simulink model "MIL_ASW"  (R2019b)
settings: Solver=FixedStepDiscrete  StartTime=0.0  StopTime=2  FixedStep=0.001  RelTol=1e-3  EnableMultiTasking=on
model workspace (MAT data in the model file):
  AccPedlCanVal : Simulink.Signal (value not decoded)
  AccPedlVal : Simulink.Signal (value not decoded)
  BrkPedlCanVal : Simulink.Signal (value not decoded)
  BrkPedlVal : Simulink.Signal (value not decoded)
  Cal1 : Simulink.Parameter (value not decoded)
  Cal10 : Simulink.Parameter (value not decoded)
  Cal11 : Simulink.Parameter (value not decoded)
  Cal12 : Simulink.Parameter (value not decoded)
  Cal2 : Simulink.Parameter (value not decoded)
  Cal3 : Simulink.Parameter (value not decoded)
  Cal4 : Simulink.Parameter (value not decoded)
  Cal5 : Simulink.Parameter (value not decoded)
  Cal6 : Simulink.Parameter (value not decoded)
  Cal7 : Simulink.Parameter (value not decoded)
  Cal8 : Simulink.Parameter (value not decoded)
  Cal9 : Simulink.Parameter (value not decoded)
  Clu1Act : Simulink.Signal (value not decoded)
  Clu1PTar : Simulink.Signal (value not decoded)
  Clu1Req : Simulink.Signal (value not decoded)
  Clu1TqTar : Simulink.Signal (value not decoded)
  Clu2Act : Simulink.Signal (value not decoded)
  Clu2PTar : Simulink.Signal (value not decoded)
  Clu2Req : Simulink.Signal (value not decoded)
  Clu2TqTar : Simulink.Signal (value not decoded)
  CluKissPtPLnch : Simulink.Parameter (value not decoded)
  CluOilTRawVal : Simulink.Signal (value not decoded)
  CluOilTVal : Simulink.Signal (value not decoded)
  CluOpenTqRatMax : Simulink.Parameter (value not decoded)
  CluPMap : Simulink.Parameter (value not decoded)
  CluPMax : Simulink.Parameter (value not decoded)
  CluPMaxGear1 : Simulink.Parameter (value not decoded)
  CluPMaxGear2 : Simulink.Parameter (value not decoded)
  CluPMaxGear3 : Simulink.Parameter (value not decoded)
  CluPMaxGear4 : Simulink.Parameter (value not decoded)
  CluPMaxGear5 : Simulink.Parameter (value not decoded)
  CluPMaxGear6 : Simulink.Parameter (value not decoded)
  CluPMaxGearR : Simulink.Parameter (value not decoded)
  CluPMin : Simulink.Parameter (value not decoded)
  CluPosnMax : Simulink.Parameter (value not decoded)
  CluSoln1IRawVal : Simulink.Signal (value not decoded)
  CluSoln1IReq : Simulink.Signal (value not decoded)
  CluSoln1IReqFlg : Simulink.Signal (value not decoded)
  CluSoln1IVal : Simulink.Signal (value not decoded)
  CluSoln1LineI : Simulink.Parameter (value not decoded)
  CluSoln1LineP : Simulink.Parameter (value not decoded)
  CluSoln1Pwm : Simulink.Signal (value not decoded)
  CluSoln2IRawVal : Simulink.Signal (value not decoded)
  CluSoln2IReq : Simulink.Signal (value not decoded)
  CluSoln2IReqFlg : Simulink.Signal (value not decoded)
  CluSoln2IVal : Simulink.Signal (value not decoded)
  CluSoln2LineI : Simulink.Parameter (value not decoded)
  CluSoln2LineP : Simulink.Parameter (value not decoded)
  CluSoln2Pwm : Simulink.Signal (value not decoded)
  CluTqMap : Simulink.Parameter (value not decoded)
  CrnkSpdRawVal : Simulink.Signal (value not decoded)
  CrnkSpdVal : Simulink.Signal (value not decoded)
  Drive_Intensity_Fuzzy : object (value not decoded)
  DrvIntenFzzy : Simulink.LookupTable (value not decoded)
  EngNIdle : Simulink.Parameter (value not decoded)
  EngNIdleMin : Simulink.Parameter (value not decoded)
  EngSpdCanVal : Simulink.Signal (value not decoded)
  EngThrCanVal : Simulink.Signal (value not decoded)
  EngTqAdd : Simulink.Parameter (value not decoded)
  EngTqCanVal : Simulink.Signal (value not decoded)
  EngTqIntvFlg : Simulink.Signal (value not decoded)
  EngTqIntvRat : Simulink.Signal (value not decoded)
  EngTqMapExtChartc : Simulink.Parameter (value not decoded)
  EngTqMapSpdIndx : Simulink.Parameter (value not decoded)
  EngTqMapThrtIndx : Simulink.Parameter (value not decoded)
  EngTqMapTqMax : Simulink.Parameter (value not decoded)
  EngTqMaxNorm : Simulink.Parameter (value not decoded)
  EngTqRef : Simulink.Parameter (value not decoded)
  EvenCluPRawVal : Simulink.Signal (value not decoded)
  EvenCluPVal : Simulink.Signal (value not decoded)
  EvenInpSpdRawVal : Simulink.Signal (value not decoded)
  EvenInpSpdVal : Simulink.Signal (value not decoded)
  FcnCallTime : Simulink.Parameter (value not decoded)
  FinalRat : Simulink.Parameter (value not decoded)
  Fork1A : Simulink.Parameter (value not decoded)
  Fork1Act : Simulink.Signal (value not decoded)
  Fork1B : Simulink.Parameter (value not decoded)
  Fork1DeltaSpdTar : Simulink.Parameter (value not decoded)
  Fork1MaxSpd1A : Simulink.Parameter (value not decoded)
  Fork1MaxSpd1B : Simulink.Parameter (value not decoded)
  Fork1MaxSpd2A : Simulink.Parameter (value not decoded)
  Fork1MaxSpd2B : Simulink.Parameter (value not decoded)
  Fork1PosnA : Simulink.Parameter (value not decoded)
  Fork1PosnB : Simulink.Parameter (value not decoded)
  Fork1PosnMaxSpd1A : Simulink.Parameter (value not decoded)
  Fork1PosnMaxSpd1B : Simulink.Parameter (value not decoded)
  Fork1PosnMaxSpd2A : Simulink.Parameter (value not decoded)
  Fork1PosnMaxSpd2B : Simulink.Parameter (value not decoded)
  Fork1PosnNeut : Simulink.Parameter (value not decoded)
  Fork1PosnNeutA : Simulink.Parameter (value not decoded)
  Fork1PosnNeutB : Simulink.Parameter (value not decoded)
  Fork1PosnRawVal : Simulink.Signal (value not decoded)
  Fork1PosnSyncA : Simulink.Parameter (value not decoded)
  Fork1PosnSyncB : Simulink.Parameter (value not decoded)
  Fork1PosnVal : Simulink.Signal (value not decoded)
  Fork1SyncTar : Simulink.Parameter (value not decoded)
  Fork2A : Simulink.Parameter (value not decoded)
  Fork2Act : Simulink.Signal (value not decoded)
  Fork2B : Simulink.Parameter (value not decoded)
  Fork2DeltaSpdTar : Simulink.Parameter (value not decoded)
  Fork2MaxSpd1A : Simulink.Parameter (value not decoded)
  Fork2MaxSpd1B : Simulink.Parameter (value not decoded)
  Fork2MaxSpd2A : Simulink.Parameter (value not decoded)
  Fork2MaxSpd2B : Simulink.Parameter (value not decoded)
  Fork2PosnA : Simulink.Parameter (value not decoded)
  Fork2PosnB : Simulink.Parameter (value not decoded)
  Fork2PosnMaxSpd1A : Simulink.Parameter (value not decoded)
  Fork2PosnMaxSpd1B : Simulink.Parameter (value not decoded)
  Fork2PosnMaxSpd2A : Simulink.Parameter (value not decoded)
  Fork2PosnMaxSpd2B : Simulink.Parameter (value not decoded)
  Fork2PosnNeut : Simulink.Parameter (value not decoded)
  Fork2PosnNeutA : Simulink.Parameter (value not decoded)
  Fork2PosnNeutB : Simulink.Parameter (value not decoded)
  Fork2PosnRawVal : Simulink.Signal (value not decoded)
  Fork2PosnSyncA : Simulink.Parameter (value not decoded)
  Fork2PosnSyncB : Simulink.Parameter (value not decoded)
  Fork2PosnVal : Simulink.Signal (value not decoded)
  Fork2SyncTar : Simulink.Parameter (value not decoded)
  Fork3A : Simulink.Parameter (value not decoded)
  Fork3Act : Simulink.Signal (value not decoded)
  Fork3B : Simulink.Parameter (value not decoded)
  Fork3DeltaSpdTar : Simulink.Parameter (value not decoded)
  Fork3MaxSpd1A : Simulink.Parameter (value not decoded)
  Fork3MaxSpd1B : Simulink.Parameter (value not decoded)
  Fork3MaxSpd2A : Simulink.Parameter (value not decoded)
  Fork3MaxSpd2B : Simulink.Parameter (value not decoded)
  Fork3PosnA : Simulink.Parameter (value not decoded)
  Fork3PosnB : Simulink.Parameter (value not decoded)
  Fork3PosnMaxSpd1A : Simulink.Parameter (value not decoded)
  Fork3PosnMaxSpd1B : Simulink.Parameter (value not decoded)
  Fork3PosnMaxSpd2A : Simulink.Parameter (value not decoded)
  Fork3PosnMaxSpd2B : Simulink.Parameter (value not decoded)
  Fork3PosnNeut : Simulink.Parameter (value not decoded)
  Fork3PosnNeutA : Simulink.Parameter (value not decoded)
  Fork3PosnNeutB : Simulink.Parameter (value not decoded)
  Fork3PosnRawVal : Simulink.Signal (value not decoded)
  Fork3PosnSyncA : Simulink.Parameter (value not decoded)
  Fork3PosnSyncB : Simulink.Parameter (value not decoded)
  Fork3PosnVal : Simulink.Signal (value not decoded)
  Fork3SyncTar : Simulink.Parameter (value not decoded)
  Fork4A : Simulink.Parameter (value not decoded)
  Fork4Act : Simulink.Signal (value not decoded)
  Fork4B : Simulink.Parameter (value not decoded)
  Fork4DeltaSpdTar : Simulink.Parameter (value not decoded)
  Fork4MaxSpd1A : Simulink.Parameter (value not decoded)
  Fork4MaxSpd1B : Simulink.Parameter (value not decoded)
  Fork4MaxSpd2A : Simulink.Parameter (value not decoded)
  Fork4MaxSpd2B : Simulink.Parameter (value not decoded)
  Fork4PosnA : Simulink.Parameter (value not decoded)
  Fork4PosnB : Simulink.Parameter (value not decoded)
  Fork4PosnMaxSpd1A : Simulink.Parameter (value not decoded)
  Fork4PosnMaxSpd1B : Simulink.Parameter (value not decoded)
  Fork4PosnMaxSpd2A : Simulink.Parameter (value not decoded)
  Fork4PosnMaxSpd2B : Simulink.Parameter (value not decoded)
  Fork4PosnNeut : Simulink.Parameter (value not decoded)
  Fork4PosnNeutA : Simulink.Parameter (value not decoded)
  Fork4PosnNeutB : Simulink.Parameter (value not decoded)
  Fork4PosnRawVal : Simulink.Signal (value not decoded)
  Fork4PosnSyncA : Simulink.Parameter (value not decoded)
  Fork4PosnSyncB : Simulink.Parameter (value not decoded)
  Fork4PosnVal : Simulink.Signal (value not decoded)
  Fork4SyncTar : Simulink.Parameter (value not decoded)
  FrntWhlRd : Simulink.Parameter (value not decoded)
  GearIdx : Simulink.Parameter (value not decoded)
  GearMax : Simulink.Parameter (value not decoded)
  GearRat : Simulink.Parameter (value not decoded)
  Launch_Engage_Fuzzy : object (value not decoded)
  LnchEngmtFzzy : Simulink.LookupTable (value not decoded)
  LubeSolnIRawVal : Simulink.Signal (value not decoded)
  LubeSolnIReq : Simulink.Signal (value not decoded)
  LubeSolnIVal : Simulink.Signal (value not decoded)
  LubeSolnLineI : Simulink.Parameter (value not decoded)
  LubeSolnLineP : Simulink.Parameter (value not decoded)
  LubeSolnPwm : Simulink.Signal (value not decoded)
  MaiLineSolnIRawVal : Simulink.Signal (value not decoded)
  MaiLineSolnIReq : Simulink.Signal (value not decoded)
  MaiLineSolnIVal : Simulink.Signal (value not decoded)
  MaiLineSolnLineI : Simulink.Parameter (value not decoded)
  MaiLineSolnLineP : Simulink.Parameter (value not decoded)
  MaiLineSolnPwm : Simulink.Signal (value not decoded)
  OddCluPRawVal : Simulink.Signal (value not decoded)
  OddCluPVal : Simulink.Signal (value not decoded)
  OddInpSpdRawVal : Simulink.Signal (value not decoded)
  OddInpSpdVal : Simulink.Signal (value not decoded)
  OutpSpdRawVal : Simulink.Signal (value not decoded)
  OutpSpdVal : Simulink.Signal (value not decoded)
  PsnsrLineP : Simulink.Parameter (value not decoded)
  PsnsrLineV : Simulink.Parameter (value not decoded)
  SftLvrCanVal : Simulink.Signal (value not decoded)
  SftLvrCfm : Simulink.Signal (value not decoded)
  SftLvrVal : Simulink.Signal (value not decoded)
  Shaft1GearAct : Simulink.Signal (value not decoded)
  Shaft1GearReq : Simulink.Signal (value not decoded)
  Shaft2GearAct : Simulink.Signal (value not decoded)
  Shaft2GearReq : Simulink.Signal (value not decoded)
  ShiftMux1SwtReq : Simulink.Signal (value not decoded)
  ShiftMux2SwtReq : Simulink.Signal (value not decoded)
  ShiftSdlEcoDwnSeln : Simulink.Parameter (value not decoded)
  ShiftSdlEcoDwnShift : Simulink.Parameter (value not decoded)
  ShiftSdlEcoUpSeln : Simulink.Parameter (value not decoded)
  ShiftSdlEcoUpShift : Simulink.Parameter (value not decoded)
  ShiftSdlPwrDwnSeln : Simulink.Parameter (value not decoded)
  ShiftSdlPwrDwnShift : Simulink.Parameter (value not decoded)
  ShiftSdlPwrUpSeln : Simulink.Parameter (value not decoded)
  ShiftSdlPwrUpShift : Simulink.Parameter (value not decoded)
  ShiftSdlSACDwnSeln : Simulink.Parameter (value not decoded)
  ShiftSdlSACDwnShift : Simulink.Parameter (value not decoded)
  ShiftSdlSACUpSeln : Simulink.Parameter (value not decoded)
  ShiftSdlSACUpShift : Simulink.Parameter (value not decoded)
  ShiftSdlThrPedlIdx : Simulink.Parameter (value not decoded)
  ShiftSoln1IRawVal : Simulink.Signal (value not decoded)
  ShiftSoln1IReq : Simulink.Signal (value not decoded)
  ShiftSoln1IVal : Simulink.Signal (value not decoded)
  ShiftSoln1LineI : Simulink.Parameter (value not decoded)
  ShiftSoln1LineP : Simulink.Parameter (value not decoded)
  ShiftSoln1Pwm : Simulink.Signal (value not decoded)
  ShiftSoln2IRawVal : Simulink.Signal (value not decoded)
  ShiftSoln2IReq : Simulink.Signal (value not decoded)
  ShiftSoln2IVal : Simulink.Signal (value not decoded)
  ShiftSoln2LineI : Simulink.Parameter (value not decoded)
  ShiftSoln2LineP : Simulink.Parameter (value not decoded)
  ShiftSoln2Pwm : Simulink.Signal (value not decoded)
  SolnOutpTRawVal : Simulink.Signal (value not decoded)
  SolnOutpTVal : Simulink.Signal (value not decoded)
  TSnsr1LineR : Simulink.Parameter (value not decoded)
  TSnsr2LineR : Simulink.Parameter (value not decoded)
  TrsmNrGearAct : Simulink.Signal (value not decoded)
  TrsmNrGearReq : Simulink.Signal (value not decoded)
  TrsmNrPreGearAct : Simulink.Signal (value not decoded)
  TrsmNrPreGearReq : Simulink.Signal (value not decoded)
  Tsnsr1LineT : Simulink.Parameter (value not decoded)
  Tsnsr2LineT : Simulink.Parameter (value not decoded)
  VehSpdCanVal : Simulink.Signal (value not decoded)
  VehSpdTrsmEstimd : Simulink.Signal (value not decoded)
  VehSpdVal : Simulink.Signal (value not decoded)
  VlvBodyTRawVal : Simulink.Signal (value not decoded)
  VlvBodyTVal : Simulink.Signal (value not decoded)
symbols that are objects in the model workspace (value not decoded): CluPMap, CluSoln1LineI, CluSoln1LineP, CluSoln2LineI, CluSoln2LineP, CluTqMap, EngNIdle, EngNIdleMin, EngTqMapThrtIndx, EngTqMapTqMax, EngTqMaxNorm, FcnCallTime, FinalRat, Fork1A, Fork1B, Fork1DeltaSpdTar, Fork1PosnA, Fork1PosnB, Fork1PosnMaxSpd1A, Fork1PosnMaxSpd1B, Fork1PosnMaxSpd2A, Fork1PosnMaxSpd2B, Fork1PosnNeut, Fork1PosnNeutA, Fork1PosnNeutB, Fork1PosnSyncA, Fork1PosnSyncB, Fork1SyncTar, Fork2A, Fork2B, Fork2DeltaSpdTar, Fork2PosnA, Fork2PosnB, Fork2PosnMaxSpd1A, Fork2PosnMaxSpd1B, Fork2PosnMaxSpd2A, Fork2PosnMaxSpd2B, Fork2PosnNeut, Fork2PosnNeutA, Fork2PosnNeutB, Fork2PosnSyncA, Fork2PosnSyncB, Fork2SyncTar, Fork3A, Fork3B, Fork3DeltaSpdTar, Fork3PosnA, Fork3PosnB, Fork3PosnMaxSpd1A, Fork3PosnMaxSpd1B, Fork3PosnMaxSpd2A, Fork3PosnMaxSpd2B, Fork3PosnNeut, Fork3PosnNeutA, Fork3PosnNeutB, Fork3PosnSyncA, Fork3PosnSyncB, Fork3SyncTar, Fork4A, Fork4B
undefined symbols (not defined in the file or in its folder): in1, out1
libraries: simulink x44, fuzblock x3
(part 3 of 10)

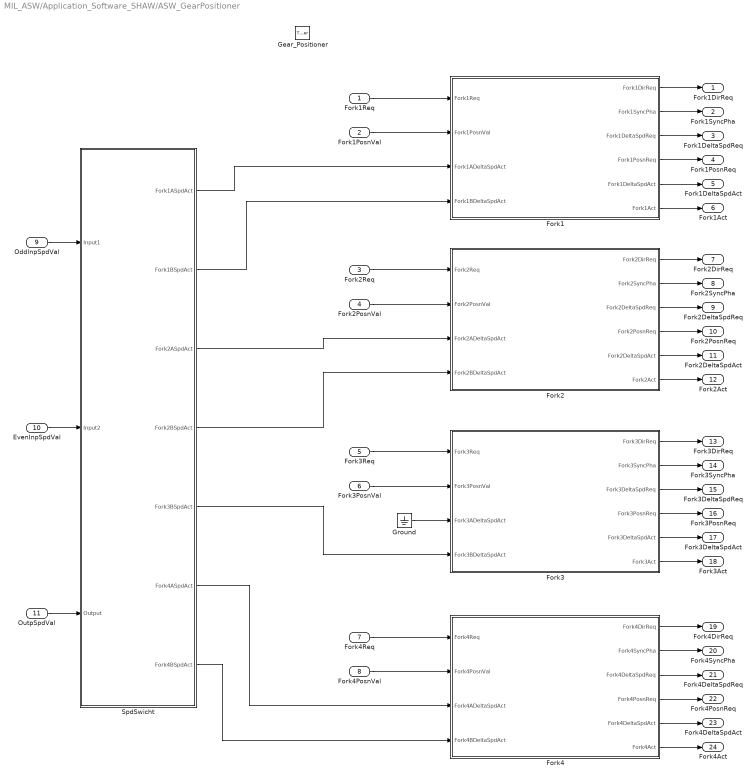
== system MIL_ASW/Application_Software_SHAW/ASW_GearPositioner ==
  Fork1Req : Inport
  Fork1PosnVal : Inport  Port=2
  Fork2Req : Inport  Port=3
  Fork2PosnVal : Inport  Port=4
  Fork3Req : Inport  Port=5
  Fork3PosnVal : Inport  Port=6
  Fork4Req : Inport  Port=7
  Fork4PosnVal : Inport  Port=8
  OddInpSpdVal : Inport  Port=9
  EvenInpSpdVal : Inport  Port=10
  OutpSpdVal : Inport  Port=11
  Gear_Positioner : TriggerPort  TriggerType=function-call  VariantControl=(inherit)  PortDimensions=1
  Fork1 : Stateflow chart  TreatAsAtomicUnit=on
  Fork2 : Stateflow chart  TreatAsAtomicUnit=on
  Fork3 : Stateflow chart  TreatAsAtomicUnit=on
  Fork4 : Stateflow chart  TreatAsAtomicUnit=on
  Ground : Ground
  SpdSwicht : Subsystem
  Fork1DirReq : Outport  VectorParamsAs1DForOutWhenUnconnected=off
  Fork1SyncPha : Outport  Port=2  VectorParamsAs1DForOutWhenUnconnected=off
  Fork1DeltaSpdReq : Outport  Port=3  VectorParamsAs1DForOutWhenUnconnected=off
  Fork1PosnReq : Outport  Port=4  VectorParamsAs1DForOutWhenUnconnected=off
  Fork1DeltaSpdAct : Outport  Port=5  VectorParamsAs1DForOutWhenUnconnected=off
  Fork1Act : Outport  Port=6  VectorParamsAs1DForOutWhenUnconnected=off
  Fork2DirReq : Outport  Port=7  VectorParamsAs1DForOutWhenUnconnected=off
  Fork2SyncPha : Outport  Port=8  VectorParamsAs1DForOutWhenUnconnected=off
  Fork2DeltaSpdReq : Outport  Port=9  VectorParamsAs1DForOutWhenUnconnected=off
  Fork2PosnReq : Outport  Port=10  VectorParamsAs1DForOutWhenUnconnected=off
  Fork2DeltaSpdAct : Outport  Port=11  VectorParamsAs1DForOutWhenUnconnected=off
  Fork2Act : Outport  Port=12  VectorParamsAs1DForOutWhenUnconnected=off
  Fork3DirReq : Outport  Port=13  VectorParamsAs1DForOutWhenUnconnected=off
  Fork3SyncPha : Outport  Port=14  VectorParamsAs1DForOutWhenUnconnected=off
  Fork3DeltaSpdReq : Outport  Port=15  VectorParamsAs1DForOutWhenUnconnected=off
  Fork3PosnReq : Outport  Port=16  VectorParamsAs1DForOutWhenUnconnected=off
  Fork3DeltaSpdAct : Outport  Port=17  VectorParamsAs1DForOutWhenUnconnected=off
  Fork3Act : Outport  Port=18  VectorParamsAs1DForOutWhenUnconnected=off
  Fork4DirReq : Outport  Port=19  VectorParamsAs1DForOutWhenUnconnected=off
  Fork4SyncPha : Outport  Port=20  VectorParamsAs1DForOutWhenUnconnected=off
  Fork4DeltaSpdReq : Outport  Port=21  VectorParamsAs1DForOutWhenUnconnected=off
  Fork4PosnReq : Outport  Port=22  VectorParamsAs1DForOutWhenUnconnected=off
  Fork4DeltaSpdAct : Outport  Port=23  VectorParamsAs1DForOutWhenUnconnected=off
  Fork4Act : Outport  Port=24  VectorParamsAs1DForOutWhenUnconnected=off
  wires:
  SpdSwicht/2(Fork1BSpdAct) -> Fork1/4(Fork1BDeltaSpdAct)
  SpdSwicht/1(Fork1ASpdAct) -> Fork1/3(Fork1ADeltaSpdAct)
  OutpSpdVal/1 -> SpdSwicht/3(Output)
  EvenInpSpdVal/1 -> SpdSwicht/2(Input2)
  OddInpSpdVal/1 -> SpdSwicht/1(Input1)
  Fork4/1(Fork4DirReq) -> Fork4DirReq/1
  Fork4PosnVal/1 -> Fork4/2(Fork4PosnVal)
  Fork4Req/1 -> Fork4/1(Fork4Req)
  Fork4/2(Fork4SyncPha) -> Fork4SyncPha/1
  Fork4/6(Fork4Act) -> Fork4Act/1
  Fork4/3(Fork4DeltaSpdReq) -> Fork4DeltaSpdReq/1
  Fork4/4(Fork4PosnReq) -> Fork4PosnReq/1
  Fork3/1(Fork3DirReq) -> Fork3DirReq/1
  Fork3PosnVal/1 -> Fork3/2(Fork3PosnVal)
  Fork3Req/1 -> Fork3/1(Fork3Req)
  Fork3/2(Fork3SyncPha) -> Fork3SyncPha/1
  Fork3/6(Fork3Act) -> Fork3Act/1
  Fork3/3(Fork3DeltaSpdReq) -> Fork3DeltaSpdReq/1
  Fork3/4(Fork3PosnReq) -> Fork3PosnReq/1
  Fork2/1(Fork2DirReq) -> Fork2DirReq/1
  Fork2PosnVal/1 -> Fork2/2(Fork2PosnVal)
  Fork2Req/1 -> Fork2/1(Fork2Req)
  Fork2/2(Fork2SyncPha) -> Fork2SyncPha/1
  Fork2/6(Fork2Act) -> Fork2Act/1
  Fork2/3(Fork2DeltaSpdReq) -> Fork2DeltaSpdReq/1
  Fork2/4(Fork2PosnReq) -> Fork2PosnReq/1
  Fork1/1(Fork1DirReq) -> Fork1DirReq/1
  Fork1PosnVal/1 -> Fork1/2(Fork1PosnVal)
  Fork1Req/1 -> Fork1/1(Fork1Req)
  Fork1/2(Fork1SyncPha) -> Fork1SyncPha/1
  Fork1/6(Fork1Act) -> Fork1Act/1
  Fork1/3(Fork1DeltaSpdReq) -> Fork1DeltaSpdReq/1
  Fork1/4(Fork1PosnReq) -> Fork1PosnReq/1
  Fork1/5(Fork1DeltaSpdAct) -> Fork1DeltaSpdAct/1
  SpdSwicht/3(Fork2ASpdAct) -> Fork2/3(Fork2ADeltaSpdAct)
  SpdSwicht/4(Fork2BSpdAct) -> Fork2/4(Fork2BDeltaSpdAct)
  Fork2/5(Fork2DeltaSpdAct) -> Fork2DeltaSpdAct/1
  SpdSwicht/5(Fork3BSpdAct) -> Fork3/4(Fork3BDeltaSpdAct)
  Fork3/5(Fork3DeltaSpdAct) -> Fork3DeltaSpdAct/1
  SpdSwicht/6(Fork4ASpdAct) -> Fork4/3(Fork4ADeltaSpdAct)
  SpdSwicht/7(Fork4BSpdAct) -> Fork4/4(Fork4BDeltaSpdAct)
  Fork4/5(Fork4DeltaSpdAct) -> Fork4DeltaSpdAct/1
  Ground/1 -> Fork3/3(Fork3ADeltaSpdAct)

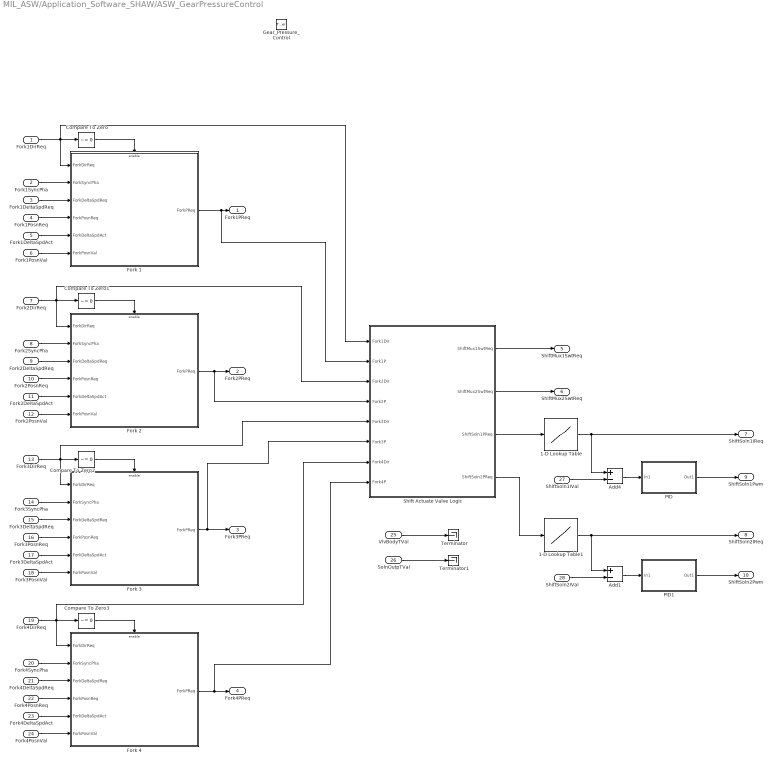
== system MIL_ASW/Application_Software_SHAW/ASW_GearPressureControl ==
  Fork1DirReq : Inport
  Fork1SyncPha : Inport  Port=2
  Fork1DeltaSpdReq : Inport  Port=3
  Fork1PosnReq : Inport  Port=4
  Fork1DeltaSpdAct : Inport  Port=5
  Fork1PosnVal : Inport  Port=6
  Fork2DirReq : Inport  Port=7
  Fork2SyncPha : Inport  Port=8
  Fork2DeltaSpdReq : Inport  Port=9
  Fork2PosnReq : Inport  Port=10
  Fork2DeltaSpdAct : Inport  Port=11
  Fork2PosnVal : Inport  Port=12
  Fork3DirReq : Inport  Port=13
  Fork3SyncPha : Inport  Port=14
  Fork3DeltaSpdReq : Inport  Port=15
  Fork3PosnReq : Inport  Port=16
  Fork3DeltaSpdAct : Inport  Port=17
  Fork3PosnVal : Inport  Port=18
  Fork4DirReq : Inport  Port=19
  Fork4SyncPha : Inport  Port=20
  Fork4DeltaSpdReq : Inport  Port=21
  Fork4PosnReq : Inport  Port=22
  Fork4DeltaSpdAct : Inport  Port=23
  Fork4PosnVal : Inport  Port=24
  VlvBodyTVal : Inport  Port=25
  SolnOutpTVal : Inport  Port=26
  ShiftSoln1IVal : Inport  Port=27
  ShiftSoln2IVal : Inport  Port=28
  Gear_Pressure_Control : TriggerPort  TriggerType=function-call  VariantControl=(inherit)  PortDimensions=1
  1-D Lookup Table : Lookup_n-D  NumberOfTableDimensions=1  BreakpointsForDimension1=ShiftSoln1LineP  BreakpointsForDimension1DataTypeStr=Inherit: Inherit from 'Breakpoint data'  Table=ShiftSoln1LineI  TableDataTypeStr=Inherit: Inherit from 'Table data'  ExtrapMethod=Clip  UseLastTableValue=on  InternalRulePriority=Speed  OutDataTypeStr=Inherit: Inherit from 'Table data'  RndMeth=Simplest  InputSameDT=on
  1-D Lookup Table1 : Lookup_n-D  NumberOfTableDimensions=1  BreakpointsForDimension1=ShiftSoln2LineP  BreakpointsForDimension1DataTypeStr=Inherit: Inherit from 'Breakpoint data'  Table=ShiftSoln2LineI  TableDataTypeStr=Inherit: Inherit from 'Table data'  ExtrapMethod=Clip  UseLastTableValue=on  InternalRulePriority=Speed  OutDataTypeStr=Inherit: Inherit from 'Table data'  RndMeth=Simplest  InputSameDT=on
  Add1 : Sum  Inputs=+-  OutDataTypeStr=int16
  Add4 : Sum  Inputs=+-  OutDataTypeStr=int16
  Compare To Zero{,1..3} (4 alike) : simulink/Logic and Bit Operations/Compare To Zero  relop=~=  OutDataTypeStr=uint8
  Fork 1 : Subsystem
  Fork 2 : Subsystem
  Fork 3 : Subsystem
  Fork 4 : Subsystem
  PID : Subsystem
  PID1 : Subsystem
  Shift Actuate Valve Logic : Stateflow chart  TreatAsAtomicUnit=on
  Terminator : Terminator
  Terminator1 : Terminator
  Fork1PReq : Outport  VectorParamsAs1DForOutWhenUnconnected=off
  Fork2PReq : Outport  Port=2  VectorParamsAs1DForOutWhenUnconnected=off
  Fork3PReq : Outport  Port=3  VectorParamsAs1DForOutWhenUnconnected=off
  Fork4PReq : Outport  Port=4  VectorParamsAs1DForOutWhenUnconnected=off
  ShiftMux1SwtReq : Outport  Port=5  VectorParamsAs1DForOutWhenUnconnected=off
  ShiftMux2SwtReq : Outport  Port=6  VectorParamsAs1DForOutWhenUnconnected=off
  ShiftSoln1IReq : Outport  Port=7  VectorParamsAs1DForOutWhenUnconnected=off
  ShiftSoln2IReq : Outport  Port=8  VectorParamsAs1DForOutWhenUnconnected=off
  ShiftSoln1Pwm : Outport  Port=9  VectorParamsAs1DForOutWhenUnconnected=off
  ShiftSoln2Pwm : Outport  Port=10  VectorParamsAs1DForOutWhenUnconnected=off
  wires:
  Fork 1/1(ForkPReq) -> Shift Actuate Valve Logic/2(Fork1P), Fork1PReq/1
  Fork1SyncPha/1 -> Fork 1/2(ForkSyncPha)
  Fork1PosnReq/1 -> Fork 1/4(ForkPosnReq)
  Fork1DeltaSpdReq/1 -> Fork 1/3(ForkDeltaSpdReq)
  Fork1PosnVal/1 -> Fork 1/6(ForkPosnVal)
  Fork1DeltaSpdAct/1 -> Fork 1/5(ForkDeltaSpdAct)
  Fork1DirReq/1 -> Fork 1/1(ForkDirReq), Shift Actuate Valve Logic/1(Fork1Dir), Compare To Zero/1
  Compare To Zero/1 -> Fork 1/Enable
  Compare To Zero1/1 -> Fork 2/Enable
  Fork2DirReq/1 -> Fork 2/1(ForkDirReq), Shift Actuate Valve Logic/3(Fork2Dir), Compare To Zero1/1
  Fork2SyncPha/1 -> Fork 2/2(ForkSyncPha)
  Fork2DeltaSpdReq/1 -> Fork 2/3(ForkDeltaSpdReq)
  Fork2PosnReq/1 -> Fork 2/4(ForkPosnReq)
  Fork2DeltaSpdAct/1 -> Fork 2/5(ForkDeltaSpdAct)
  Fork2PosnVal/1 -> Fork 2/6(ForkPosnVal)
  Fork 2/1(ForkPReq) -> Shift Actuate Valve Logic/4(Fork2P), Fork2PReq/1
  Compare To Zero2/1 -> Fork 3/Enable
  Fork 3/1(ForkPReq) -> Shift Actuate Valve Logic/6(Fork3P), Fork3PReq/1
  Compare To Zero3/1 -> Fork 4/Enable
  Fork3DirReq/1 -> Fork 3/1(ForkDirReq), Shift Actuate Valve Logic/5(Fork3Dir), Compare To Zero2/1
  Fork3PosnReq/1 -> Fork 3/4(ForkPosnReq)
  Fork3SyncPha/1 -> Fork 3/2(ForkSyncPha)
  Fork3DeltaSpdAct/1 -> Fork 3/5(ForkDeltaSpdAct)
  Fork3PosnVal/1 -> Fork 3/6(ForkPosnVal)
  Fork3DeltaSpdReq/1 -> Fork 3/3(ForkDeltaSpdReq)
  Fork4DirReq/1 -> Fork 4/1(ForkDirReq), Shift Actuate Valve Logic/7(Fork4Dir), Compare To Zero3/1
  Fork4PosnVal/1 -> Fork 4/6(ForkPosnVal)
  Fork4DeltaSpdAct/1 -> Fork 4/5(ForkDeltaSpdAct)
  Fork4PosnReq/1 -> Fork 4/4(ForkPosnReq)
  Fork4DeltaSpdReq/1 -> Fork 4/3(ForkDeltaSpdReq)
  Fork4SyncPha/1 -> Fork 4/2(ForkSyncPha)
  Fork 4/1(ForkPReq) -> Shift Actuate Valve Logic/8(Fork4P), Fork4PReq/1
  Shift Actuate Valve Logic/1(ShiftMux1SwtReq) -> ShiftMux1SwtReq/1
  Shift Actuate Valve Logic/2(ShiftMux2SwtReq) -> ShiftMux2SwtReq/1
  VlvBodyTVal/1 -> Terminator/1
  SolnOutpTVal/1 -> Terminator1/1
  Shift Actuate Valve Logic/3(ShiftSoln1PReq) -> 1-D Lookup Table/1
  Shift Actuate Valve Logic/4(ShiftSoln2PReq) -> 1-D Lookup Table1/1
  1-D Lookup Table/1 -> Add4/1, ShiftSoln1IReq/1
  Add4/1 -> PID/1(In1)
  ShiftSoln1IVal/1 -> Add4/2
  1-D Lookup Table1/1 -> Add1/1, ShiftSoln2IReq/1
  Add1/1 -> PID1/1(In1)
  ShiftSoln2IVal/1 -> Add1/2
  PID1/1(Out1) -> ShiftSoln2Pwm/1
  PID/1(Out1) -> ShiftSoln1Pwm/1

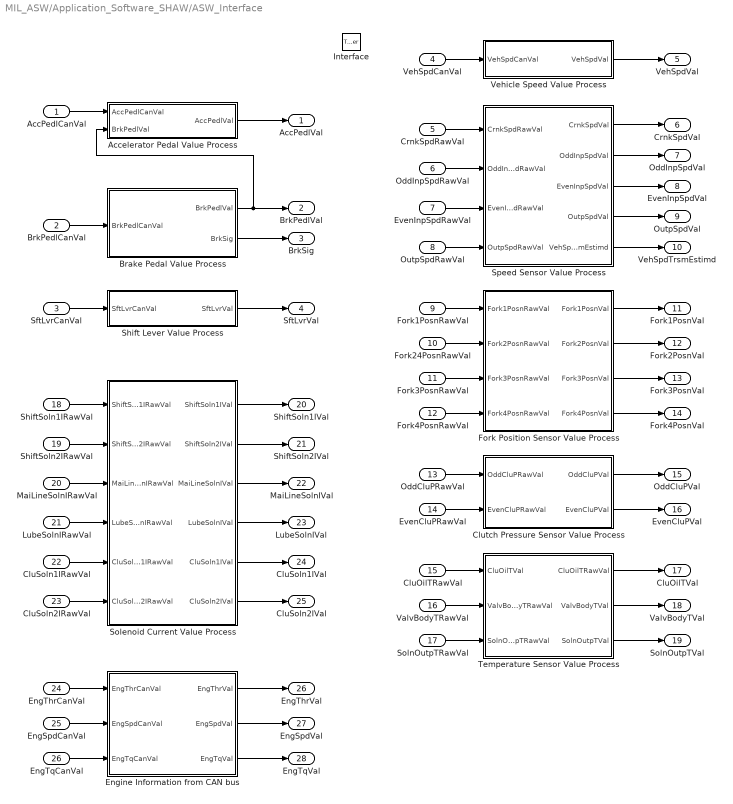
== system MIL_ASW/Application_Software_SHAW/ASW_Interface ==
  AccPedlCanVal : Inport
  BrkPedlCanVal : Inport  Port=2
  SftLvrCanVal : Inport  Port=3
  VehSpdCanVal : Inport  Port=4
  CrnkSpdRawVal : Inport  Port=5
  OddInpSpdRawVal : Inport  Port=6
  EvenInpSpdRawVal : Inport  Port=7
  OutpSpdRawVal : Inport  Port=8
  Fork1PosnRawVal : Inport  Port=9
  Fork24PosnRawVal : Inport  Port=10
  Fork3PosnRawVal : Inport  Port=11
  Fork4PosnRawVal : Inport  Port=12
  OddCluPRawVal : Inport  Port=13
  EvenCluPRawVal : Inport  Port=14
  CluOilTRawVal : Inport  Port=15
  ValvBodyTRawVal : Inport  Port=16
  SolnOutpTRawVal : Inport  Port=17
  ShiftSoln1IRawVal : Inport  Port=18
  ShiftSoln2IRawVal : Inport  Port=19
  MaiLineSolnIRawVal : Inport  Port=20
  LubeSolnIRawVal : Inport  Port=21
  CluSoln1IRawVal : Inport  Port=22
  CluSoln2IRawVal : Inport  Port=23
  EngThrCanVal : Inport  Port=24
  EngSpdCanVal : Inport  Port=25
  EngTqCanVal : Inport  Port=26
  Interface : TriggerPort  TriggerType=function-call  VariantControl=(inherit)  PortDimensions=1
  Accelerator Pedal Value Process : Subsystem  TreatAsAtomicUnit=on
  Brake Pedal Value Process : Subsystem  TreatAsAtomicUnit=on
  Clutch Pressure Sensor Value Process : Subsystem  TreatAsAtomicUnit=on
  Engine Information from CAN bus : Subsystem  TreatAsAtomicUnit=on
  Fork Position Sensor Value Process : Subsystem  TreatAsAtomicUnit=on
  Shift Lever Value Process : Subsystem  TreatAsAtomicUnit=on
  Solenoid Current Value Process : Subsystem  TreatAsAtomicUnit=on
  Speed Sensor Value Process : Subsystem  TreatAsAtomicUnit=on
  Temperature Sensor Value Process : Subsystem  TreatAsAtomicUnit=on
  Vehicle Speed Value Process : Subsystem  TreatAsAtomicUnit=on
  AccPedlVal : Outport  VectorParamsAs1DForOutWhenUnconnected=off
  BrkPedlVal : Outport  Port=2  OutDataTypeStr=uint8  VectorParamsAs1DForOutWhenUnconnected=off
  BrkSig : Outport  Port=3  OutDataTypeStr=uint8  VectorParamsAs1DForOutWhenUnconnected=off
  SftLvrVal : Outport  Port=4  OutDataTypeStr=uint8  VectorParamsAs1DForOutWhenUnconnected=off
  VehSpdVal : Outport  Port=5  VectorParamsAs1DForOutWhenUnconnected=off
  CrnkSpdVal : Outport  Port=6  VectorParamsAs1DForOutWhenUnconnected=off
  OddInpSpdVal : Outport  Port=7  VectorParamsAs1DForOutWhenUnconnected=off
  EvenInpSpdVal : Outport  Port=8  VectorParamsAs1DForOutWhenUnconnected=off
  OutpSpdVal : Outport  Port=9  VectorParamsAs1DForOutWhenUnconnected=off
  VehSpdTrsmEstimd : Outport  Port=10  VectorParamsAs1DForOutWhenUnconnected=off
  Fork1PosnVal : Outport  Port=11  VectorParamsAs1DForOutWhenUnconnected=off
  Fork2PosnVal : Outport  Port=12  VectorParamsAs1DForOutWhenUnconnected=off
  Fork3PosnVal : Outport  Port=13  VectorParamsAs1DForOutWhenUnconnected=off
  Fork4PosnVal : Outport  Port=14  VectorParamsAs1DForOutWhenUnconnected=off
  OddCluPVal : Outport  Port=15  VectorParamsAs1DForOutWhenUnconnected=off
  EvenCluPVal : Outport  Port=16  VectorParamsAs1DForOutWhenUnconnected=off
  CluOilTVal : Outport  Port=17  VectorParamsAs1DForOutWhenUnconnected=off
  ValvBodyTVal : Outport  Port=18  VectorParamsAs1DForOutWhenUnconnected=off
  SolnOutpTVal : Outport  Port=19  VectorParamsAs1DForOutWhenUnconnected=off
  ShiftSoln1IVal : Outport  Port=20  VectorParamsAs1DForOutWhenUnconnected=off
  ShiftSoln2IVal : Outport  Port=21  VectorParamsAs1DForOutWhenUnconnected=off
  MaiLineSolnIVal : Outport  Port=22  VectorParamsAs1DForOutWhenUnconnected=off
  LubeSolnIVal : Outport  Port=23  VectorParamsAs1DForOutWhenUnconnected=off
  CluSoln1IVal : Outport  Port=24  VectorParamsAs1DForOutWhenUnconnected=off
  CluSoln2IVal : Outport  Port=25  VectorParamsAs1DForOutWhenUnconnected=off
  EngThrVal : Outport  Port=26  VectorParamsAs1DForOutWhenUnconnected=off
  EngSpdVal : Outport  Port=27  VectorParamsAs1DForOutWhenUnconnected=off
  EngTqVal : Outport  Port=28  VectorParamsAs1DForOutWhenUnconnected=off
  wires:
  Accelerator Pedal Value Process/1(AccPedlVal) -> AccPedlVal/1
  Shift Lever Value Process/1(SftLvrVal) -> SftLvrVal/1
  Brake Pedal Value Process/1(BrkPedlVal) -> Accelerator Pedal Value Process/2(BrkPedlVal), BrkPedlVal/1
  BrkPedlCanVal/1 -> Brake Pedal Value Process/1(BrkPedlCanVal)
  SftLvrCanVal/1 -> Shift Lever Value Process/1(SftLvrCanVal)
  AccPedlCanVal/1 -> Accelerator Pedal Value Process/1(AccPedlCanVal)
  VehSpdCanVal/1 -> Vehicle Speed Value Process/1(VehSpdCanVal)
  Vehicle Speed Value Process/1(VehSpdVal) -> VehSpdVal/1
  CrnkSpdRawVal/1 -> Speed Sensor Value Process/1(CrnkSpdRawVal)
  Speed Sensor Value Process/1(CrnkSpdVal) -> CrnkSpdVal/1
  OddInpSpdRawVal/1 -> Speed Sensor Value Process/2(OddInpSpdRawVal)
  EvenInpSpdRawVal/1 -> Speed Sensor Value Process/3(EvenInpSpdRawVal)
  OutpSpdRawVal/1 -> Speed Sensor Value Process/4(OutpSpdRawVal)
  Speed Sensor Value Process/2(OddInpSpdVal) -> OddInpSpdVal/1
  Speed Sensor Value Process/3(EvenInpSpdVal) -> EvenInpSpdVal/1
  Speed Sensor Value Process/4(OutpSpdVal) -> OutpSpdVal/1
  Fork1PosnRawVal/1 -> Fork Position Sensor Value Process/1(Fork1PosnRawVal)
  Fork4PosnRawVal/1 -> Fork Position Sensor Value Process/4(Fork4PosnRawVal)
  Fork3PosnRawVal/1 -> Fork Position Sensor Value Process/3(Fork3PosnRawVal)
  Fork24PosnRawVal/1 -> Fork Position Sensor Value Process/2(Fork2PosnRawVal)
  Fork Position Sensor Value Process/1(Fork1PosnVal) -> Fork1PosnVal/1
  Fork Position Sensor Value Process/2(Fork2PosnVal) -> Fork2PosnVal/1
  Fork Position Sensor Value Process/3(Fork3PosnVal) -> Fork3PosnVal/1
  Fork Position Sensor Value Process/4(Fork4PosnVal) -> Fork4PosnVal/1
  EvenCluPRawVal/1 -> Clutch Pressure Sensor Value Process/2(EvenCluPRawVal)
  OddCluPRawVal/1 -> Clutch Pressure Sensor Value Process/1(OddCluPRawVal)
  Clutch Pressure Sensor Value Process/1(OddCluPVal) -> OddCluPVal/1
  CluOilTRawVal/1 -> Temperature Sensor Value Process/1(CluOilTVal)
  ValvBodyTRawVal/1 -> Temperature Sensor Value Process/2(ValvBodyTRawVal)
  SolnOutpTRawVal/1 -> Temperature Sensor Value Process/3(SolnOutpTRawVal)
  Temperature Sensor Value Process/1(CluOilTRawVal) -> CluOilTVal/1
  Temperature Sensor Value Process/2(ValvBodyTVal) -> ValvBodyTVal/1
  Temperature Sensor Value Process/3(SolnOutpTVal) -> SolnOutpTVal/1
  Speed Sensor Value Process/5(VehSpdTrsmEstimd) -> VehSpdTrsmEstimd/1
  Brake Pedal Value Process/2(BrkSig) -> BrkSig/1
  ShiftSoln1IRawVal/1 -> Solenoid Current Value Process/1(ShiftSoln1IRawVal)
  Solenoid Current Value Process/1(ShiftSoln1IVal) -> ShiftSoln1IVal/1
  Solenoid Current Value Process/2(ShiftSoln2IVal) -> ShiftSoln2IVal/1
  Solenoid Current Value Process/3(MaiLineSolnIVal) -> MaiLineSolnIVal/1
  Solenoid Current Value Process/4(LubeSolnIVal) -> LubeSolnIVal/1
  Solenoid Current Value Process/5(CluSoln1IVal) -> CluSoln1IVal/1
  Solenoid Current Value Process/6(CluSoln2IVal) -> CluSoln2IVal/1
  ShiftSoln2IRawVal/1 -> Solenoid Current Value Process/2(ShiftSoln2IRawVal)
  MaiLineSolnIRawVal/1 -> Solenoid Current Value Process/3(MaiLineSolnIRawVal)
  LubeSolnIRawVal/1 -> Solenoid Current Value Process/4(LubeSolnIRawVal)
  CluSoln1IRawVal/1 -> Solenoid Current Value Process/5(CluSoln1IRawVal)
  CluSoln2IRawVal/1 -> Solenoid Current Value Process/6(CluSoln2IRawVal)
  Clutch Pressure Sensor Value Process/2(EvenCluPVal) -> EvenCluPVal/1
  EngThrCanVal/1 -> Engine Information from CAN bus/1(EngThrCanVal)
  EngTqCanVal/1 -> Engine Information from CAN bus/3(EngTqCanVal)
  Engine Information from CAN bus/3(EngTqVal) -> EngTqVal/1
  Engine Information from CAN bus/2(EngSpdVal) -> EngSpdVal/1
  EngSpdCanVal/1 -> Engine Information from CAN bus/2(EngSpdCanVal)
  Engine Information from CAN bus/1(EngThrVal) -> EngThrVal/1

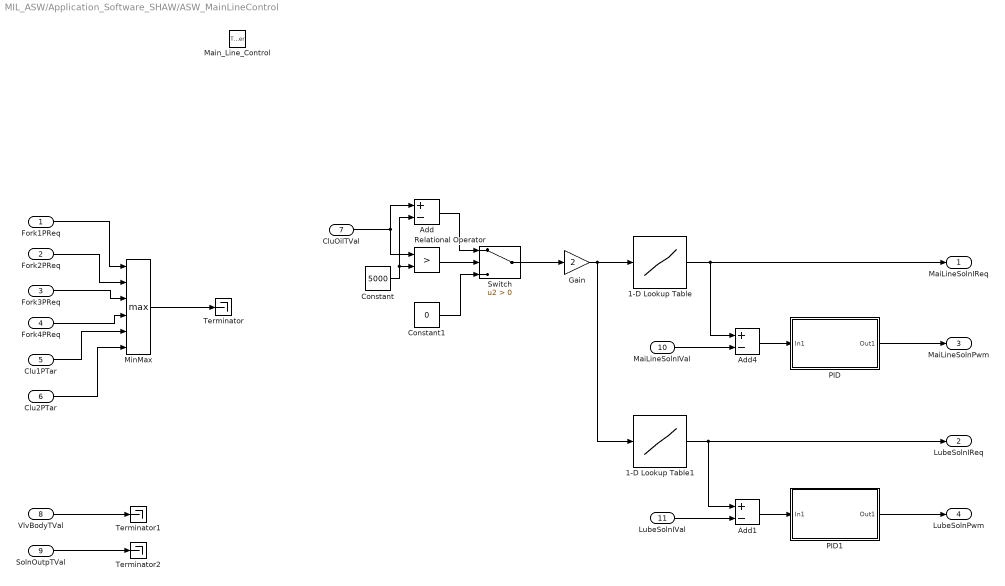
== system MIL_ASW/Application_Software_SHAW/ASW_MainLineControl ==
  Fork1PReq : Inport
  Fork2PReq : Inport  Port=2
  Fork3PReq : Inport  Port=3
  Fork4PReq : Inport  Port=4
  Clu1PTar : Inport  Port=5
  Clu2PTar : Inport  Port=6
  CluOilTVal : Inport  Port=7
  VlvBodyTVal : Inport  Port=8
  SolnOutpTVal : Inport  Port=9
  MaiLineSolnIVal : Inport  Port=10
  LubeSolnIVal : Inport  Port=11
  Main_Line_Control : TriggerPort  TriggerType=function-call  VariantControl=(inherit)  PortDimensions=1
  1-D Lookup Table : Lookup_n-D  NumberOfTableDimensions=1  BreakpointsForDimension1=MaiLineSolnLineP  BreakpointsForDimension1DataTypeStr=Inherit: Inherit from 'Breakpoint data'  Table=MaiLineSolnLineI  TableDataTypeStr=Inherit: Inherit from 'Table data'  ExtrapMethod=Clip  InternalRulePriority=Speed  OutDataTypeStr=Inherit: Inherit from 'Table data'  RndMeth=Simplest  InputSameDT=on
  1-D Lookup Table1 : Lookup_n-D  NumberOfTableDimensions=1  BreakpointsForDimension1=LubeSolnLineP  BreakpointsForDimension1DataTypeStr=Inherit: Inherit from 'Breakpoint data'  Table=LubeSolnLineI  TableDataTypeStr=Inherit: Inherit from 'Table data'  ExtrapMethod=Clip  InternalRulePriority=Speed  OutDataTypeStr=Inherit: Inherit from 'Table data'  RndMeth=Simplest  InputSameDT=on
  Add : Sum  Inputs=+-  OutDataTypeStr=uint16
  Add1 : Sum  Inputs=+-  OutDataTypeStr=int16
  Add4 : Sum  Inputs=+-  OutDataTypeStr=int16
  Constant : Constant  Value=5000  OutDataTypeStr=uint16
  Constant1 : Constant  Value=0  OutDataTypeStr=uint16
  Gain : Gain  Gain=2  OutDataTypeStr=uint16
  MinMax : MinMax  Function=max  Inputs=6  OutDataTypeStr=uint16
  PID : Subsystem
  PID1 : Subsystem
  Relational Operator : RelationalOperator  Operator=>  OutDataTypeStr=boolean  RndMeth=Nearest
  Switch : Switch  Criteria=u2 > Threshold  OutDataTypeStr=uint16
  Terminator : Terminator
  Terminator1 : Terminator
  Terminator2 : Terminator
  MaiLineSolnIReq : Outport  VectorParamsAs1DForOutWhenUnconnected=off
  LubeSolnIReq : Outport  Port=2  VectorParamsAs1DForOutWhenUnconnected=off
  MaiLineSolnPwm : Outport  Port=3  VectorParamsAs1DForOutWhenUnconnected=off
  LubeSolnPwm : Outport  Port=4  VectorParamsAs1DForOutWhenUnconnected=off
  wires:
  Fork2PReq/1 -> MinMax/2
  Fork1PReq/1 -> MinMax/1
  Fork3PReq/1 -> MinMax/3
  Fork4PReq/1 -> MinMax/4
  Clu1PTar/1 -> MinMax/5
  Clu2PTar/1 -> MinMax/6
  MinMax/1 -> Terminator/1
  VlvBodyTVal/1 -> Terminator1/1
  SolnOutpTVal/1 -> Terminator2/1
  CluOilTVal/1 -> Relational Operator/1, Add/1
  Constant/1 -> Add/2, Relational Operator/2
  Relational Operator/1 -> Switch/2
  Add/1 -> Switch/1
  Constant1/1 -> Switch/3
  Switch/1 -> Gain/1
  Gain/1 -> 1-D Lookup Table1/1, 1-D Lookup Table/1
  1-D Lookup Table/1 -> Add4/1, MaiLineSolnIReq/1
  Add4/1 -> PID/1(In1)
  MaiLineSolnIVal/1 -> Add4/2
  PID/1(Out1) -> MaiLineSolnPwm/1
  1-D Lookup Table1/1 -> Add1/1, LubeSolnIReq/1
  Add1/1 -> PID1/1(In1)
  LubeSolnIVal/1 -> Add1/2
  PID1/1(Out1) -> LubeSolnPwm/1

== system MIL_ASW/Application_Software_SHAW/ASW_ShaftAccessControl ==
  "TrsmNrPreGearReq " : Inport
  "TrsmNrGearReq " : Inport  Port=2
  "Shaft1GearAct " : Inport  Port=3
  "Shaft2GearAct " : Inport  Port=4
  "Clu1Act " : Inport  Port=5
  "Clu2Act " : Inport  Port=6
  BrkSig : Inport  Port=7
  SftLvrVal : Inport  Port=8
  Shaft_Access_Control : TriggerPort  TriggerType=function-call  VariantControl=(inherit)  PortDimensions=1
  Chart1 : Stateflow chart  TreatAsAtomicUnit=on
  Shift lever match to gear : Subsystem
  Shaft1GearReq : Outport  VectorParamsAs1DForOutWhenUnconnected=off
  Shaft2GearReq : Outport  Port=2  VectorParamsAs1DForOutWhenUnconnected=off
  Clu1Req : Outport  Port=3  VectorParamsAs1DForOutWhenUnconnected=off
  Clu2Req : Outport  Port=4  VectorParamsAs1DForOutWhenUnconnected=off
  TrsmNrGearAct : Outport  Port=5  VectorParamsAs1DForOutWhenUnconnected=off
  TrsmNrPreGearAct : Outport  Port=6  VectorParamsAs1DForOutWhenUnconnected=off
  TrsmNrGearErr : Outport  Port=7  VectorParamsAs1DForOutWhenUnconnected=off
  TrsmNrPreGearErr : Outport  Port=8  VectorParamsAs1DForOutWhenUnconnected=off
  SftLvrCfm : Outport  Port=9  VectorParamsAs1DForOutWhenUnconnected=off
  wires:
  Chart1/7(TrsmNrGearErr) -> TrsmNrGearErr/1
  Chart1/2(Shaft2GearReq) -> Shaft2GearReq/1
  Chart1/1(Shaft1GearReq) -> Shaft1GearReq/1
  "TrsmNrPreGearReq "/1 -> Chart1/1(TrsmNrPreGearReq)
  "Shaft1GearAct "/1 -> Chart1/3(Shaft1GearAct)
  "Clu1Act "/1 -> Chart1/5(Clu1Act)
  "Clu2Act "/1 -> Chart1/6(Clu2Act)
  Chart1/8(TrsmNrPreGearErr) -> TrsmNrPreGearErr/1
  BrkSig/1 -> Chart1/7(BrkSig)
  Chart1/6(TrsmNrPreGearAct) -> Shift lever match to gear/3(TrsmNrPreGearAct), TrsmNrPreGearAct/1
  Chart1/5(TrsmNrGearAct) -> Shift lever match to gear/2(TrsmNrGearAct), TrsmNrGearAct/1
  SftLvrVal/1 -> Shift lever match to gear/1(SftLvrVal)
  Shift lever match to gear/1(SftLvrCfm) -> SftLvrCfm/1
  Chart1/3(Clu1Req) -> Clu1Req/1
  Chart1/4(Clu2Req) -> Clu2Req/1
  "TrsmNrGearReq "/1 -> Chart1/2(TrsmNrGearReq)
  "Shaft2GearAct "/1 -> Chart1/4(Shaft2GearAct)

== system MIL_ASW/Application_Software_SHAW/ASW_ShaftControl ==
  Shaft1GearReq : Inport
  Shaft2GearReq : Inport  Port=2
  Fork1Act : Inport  Port=3  OutDataTypeStr=uint8
  Fork2Act : Inport  Port=4
  Fork3Act : Inport  Port=5
  Fork4Act : Inport  Port=6
  Shaft_Control : TriggerPort  TriggerType=function-call  VariantControl=(inherit)  PortDimensions=1
  Even Part : Stateflow chart  TreatAsAtomicUnit=on
  Odd Part : Stateflow chart  TreatAsAtomicUnit=on
  Shaft1GearAct : Outport  VectorParamsAs1DForOutWhenUnconnected=off
  Shaft2GearAct : Outport  Port=2  VectorParamsAs1DForOutWhenUnconnected=off
  Fork1Req : Outport  Port=3  VectorParamsAs1DForOutWhenUnconnected=off
  Fork2Req : Outport  Port=4  VectorParamsAs1DForOutWhenUnconnected=off
  Fork3Req : Outport  Port=5  VectorParamsAs1DForOutWhenUnconnected=off
  Fork4Req : Outport  Port=6  VectorParamsAs1DForOutWhenUnconnected=off
  Shaft1GearErr : Outport  Port=7  VectorParamsAs1DForOutWhenUnconnected=off
  Shaft2GearErr : Outport  Port=8  VectorParamsAs1DForOutWhenUnconnected=off
  wires:
  Shaft2GearReq/1 -> Even Part/3(Shaft2GearReq)
  Even Part/1(Fork2Req) -> Fork2Req/1
  Even Part/2(Fork4Req) -> Fork4Req/1
  Fork2Act/1 -> Even Part/1(Fork2Act)
  Fork4Act/1 -> Even Part/2(Fork4Act)
  Even Part/3(Shaft2GearAct) -> Shaft2GearAct/1
  Even Part/4(Shaft2GearErr) -> Shaft2GearErr/1
  Odd Part/4(Shaft1GearErr) -> Shaft1GearErr/1
  Odd Part/3(Shaft1GearAct) -> Shaft1GearAct/1
  Fork3Act/1 -> Odd Part/2(Fork3Act)
  Fork1Act/1 -> Odd Part/1(Fork1Act)
  Odd Part/2(Fork3Req) -> Fork3Req/1
  Odd Part/1(Fork1Req) -> Fork1Req/1
  Shaft1GearReq/1 -> Odd Part/3(Shaft1GearReq)

== system MIL_ASW/Application_Software_SHAW/ASW_TorqueControl ==
  Clu1TqTar : Inport  OutDataTypeStr=uint16
  Clu2TqTar : Inport  Port=2  OutDataTypeStr=uint16
  Clu1PAct : Inport  Port=3
  Clu2PAct : Inport  Port=4
  EngN : Inport  Port=5  OutDataTypeStr=uint16
  InpShaft1N : Inport  Port=6  OutDataTypeStr=uint16
  InpShaft2N : Inport  Port=7
  CluT : Inport  Port=8
  Torque_Control : TriggerPort  TriggerType=function-call  VariantControl=(inherit)  PortDimensions=1
  1-D Lookup Table1 : Lookup_n-D  NumberOfTableDimensions=1  BreakpointsForDimension1=CluTqMap  BreakpointsForDimension1DataTypeStr=Inherit: Inherit from 'Breakpoint data'  Table=CluPMap  TableDataTypeStr=Inherit: Inherit from 'Table data'  ExtrapMethod=Clip  UseLastTableValue=on  OutDataTypeStr=Inherit: Inherit from 'Table data'  RndMeth=Simplest  InputSameDT=on
  1-D Lookup Table2 : Lookup_n-D  NumberOfTableDimensions=1  BreakpointsForDimension1=CluTqMap  BreakpointsForDimension1DataTypeStr=Inherit: Inherit from 'Breakpoint data'  Table=CluPMap  TableDataTypeStr=Inherit: Inherit from 'Table data'  ExtrapMethod=Clip  UseLastTableValue=on  OutDataTypeStr=Inherit: Inherit from 'Table data'  RndMeth=Simplest  InputSameDT=on
  1-D Lookup Table3 : Lookup_n-D  NumberOfTableDimensions=1  BreakpointsForDimension1=CluPMap  BreakpointsForDimension1DataTypeStr=Inherit: Inherit from 'Breakpoint data'  Table=CluTqMap  TableDataTypeStr=Inherit: Inherit from 'Table data'  ExtrapMethod=Clip  UseLastTableValue=on  OutDataTypeStr=Inherit: Inherit from 'Table data'  RndMeth=Simplest  InputSameDT=on
  1-D Lookup Table4 : Lookup_n-D  NumberOfTableDimensions=1  BreakpointsForDimension1=CluPMap  BreakpointsForDimension1DataTypeStr=Inherit: Inherit from 'Breakpoint data'  Table=CluTqMap  TableDataTypeStr=Inherit: Inherit from 'Table data'  ExtrapMethod=Clip  UseLastTableValue=on  OutDataTypeStr=Inherit: Inherit from 'Table data'  RndMeth=Simplest  InputSameDT=on
  Add : Sum  Inputs=+-  OutDataTypeStr=int16
  Add1 : Sum  Inputs=+-  OutDataTypeStr=int16
  Terminator : Terminator
  Terminator1 : Terminator
  Terminator2 : Terminator
  Clu1PTar : Outport  OutDataTypeStr=uint16  VectorParamsAs1DForOutWhenUnconnected=off
  Clu2PTar : Outport  Port=2  OutDataTypeStr=uint16  VectorParamsAs1DForOutWhenUnconnected=off
  Clu1TqCpEstimd : Outport  Port=3  VectorParamsAs1DForOutWhenUnconnected=off
  Clu2TqCpEstimd : Outport  Port=4  VectorParamsAs1DForOutWhenUnconnected=off
  wires:
  EngN/1 -> Add1/1, Add/1
  InpShaft1N/1 -> Add/2
  InpShaft2N/1 -> Add1/2
  Add/1 -> Terminator/1
  Add1/1 -> Terminator1/1
  CluT/1 -> Terminator2/1
  Clu1TqTar/1 -> 1-D Lookup Table1/1
  Clu2TqTar/1 -> 1-D Lookup Table2/1
  1-D Lookup Table1/1 -> Clu1PTar/1
  1-D Lookup Table2/1 -> Clu2PTar/1
  1-D Lookup Table4/1 -> Clu2TqCpEstimd/1
  Clu2PAct/1 -> 1-D Lookup Table4/1
  1-D Lookup Table3/1 -> Clu1TqCpEstimd/1
  Clu1PAct/1 -> 1-D Lookup Table3/1

== system MIL_ASW/Application_Software_SHAW/TR_Scheduler ==
  Scheduler : Stateflow chart  TreatAsAtomicUnit=on
  Fncall_If : Outport  VectorParamsAs1DForOutWhenUnconnected=off
  Fncall_DrvgStgy : Outport  Port=2  VectorParamsAs1DForOutWhenUnconnected=off
  Fncall_ShaftAcsCtrl : Outport  Port=3  VectorParamsAs1DForOutWhenUnconnected=off
  Fncall_ShaftCtrl : Outport  Port=4  VectorParamsAs1DForOutWhenUnconnected=off
  Fncall_GearPosnr : Outport  Port=5  VectorParamsAs1DForOutWhenUnconnected=off
  Fncall_GearPCtrl : Outport  Port=6  VectorParamsAs1DForOutWhenUnconnected=off
  Fncall_CluCtrl : Outport  Port=7  VectorParamsAs1DForOutWhenUnconnected=off
  Fncall_CluPCtrl : Outport  Port=8  VectorParamsAs1DForOutWhenUnconnected=off
  Fncall_TqCtrl : Outport  Port=9  VectorParamsAs1DForOutWhenUnconnected=off
  Fncall_MaiLineCtrl : Outport  Port=10  VectorParamsAs1DForOutWhenUnconnected=off
  wires:
  Scheduler/1(Fncall_If()) -> Fncall_If/1
  Scheduler/2(Fncall_DrvgStgy()) -> Fncall_DrvgStgy/1
  Scheduler/3(Fncall_ShaftAcsCtrl()) -> Fncall_ShaftAcsCtrl/1
  Scheduler/4(Fncall_ShaftCtrl()) -> Fncall_ShaftCtrl/1
  Scheduler/5(Fncall_GearPosnr()) -> Fncall_GearPosnr/1
  Scheduler/6(Fncall_GearPCtrl()) -> Fncall_GearPCtrl/1
  Scheduler/7(Fncall_CluCtrl()) -> Fncall_CluCtrl/1
  Scheduler/8(Fncall_CluPCtrl()) -> Fncall_CluPCtrl/1
  Scheduler/9(Fncall_TqCtrl()) -> Fncall_TqCtrl/1
  Scheduler/10(Fncall_MaiLineCtrl()) -> Fncall_MaiLineCtrl/1

== system MIL_ASW/Application_Software_SHAW/ASW_ClutchControl_new/Clutch_Control_Strategy/Close_Torque_Target ==
  EngThr : Inport  OutDataTypeStr=uint8  PortDimensions=1
  f : TriggerPort  TriggerType=function-call  VariantControl=(inherit)
      settings: CopyFcn=Stateflow.SLINSF.SimulinkMan.removeBlockPreDeleteFcn  PreDeleteFcn=Stateflow.SLINSF.SimulinkMan.unsafePredeleteFcn
  1-D Lookup Table : Lookup_n-D  NumberOfTableDimensions=1  BreakpointsForDimension1=EngTqMapThrtIndx  BreakpointsForDimension1DataTypeStr=Inherit: Inherit from 'Breakpoint data'  Table=EngTqMapTqMax  TableDataTypeStr=Inherit: Inherit from 'Table data'  ExtrapMethod=Clip  UseLastTableValue=on  OutDataTypeStr=Inherit: Inherit from 'Table data'  RndMeth=Simplest  InputSameDT=on
  Gain : Gain  Gain=6/5  OutDataTypeStr=uint16
  Tq : Outport  OutDataTypeStr=uint16  PortDimensions=1  VectorParamsAs1DForOutWhenUnconnected=off
  wires:
  1-D Lookup Table/1 -> Gain/1
  EngThr/1 -> 1-D Lookup Table/1
  Gain/1 -> Tq/1

== system MIL_ASW/Application_Software_SHAW/ASW_ClutchControl_new/Clutch_Control_Strategy/Driver_Intention_Fuzzy ==
  AccPeld : Inport  OutDataTypeStr=uint8  PortDimensions=1
  f : TriggerPort  TriggerType=function-call  VariantControl=(inherit)
      settings: CopyFcn=Stateflow.SLINSF.SimulinkMan.removeBlockPreDeleteFcn  PreDeleteFcn=Stateflow.SLINSF.SimulinkMan.unsafePredeleteFcn
  Constant1 : Constant  Value=100  OutDataTypeStr=int16
  Constant2 : Constant  Value=FcnCallTime  OutDataTypeStr=uint8
  Constant3 : Constant  Value=1000  OutDataTypeStr=int16
  Divide : Product  Inputs=*/  OutDataTypeStr=int16
  Divide1 : Product  Inputs=*/  OutDataTypeStr=int16
  Fuzzy Logic Controller : fuzblock/Fuzzy Logic  Controller  FIS='Launch_Intensity_Fuzzy.fis'  OutputSampleNumber=101  DataType=single  FuzzifiedInputs=off  RuleFiringStrengths=off  RuleOutputs=off  AggregatedOutputs=off  SimulateUsing=Code generation  OutOfRangeInputValueMessage=warning  NoRuleFiredMessage=warning  EmptyOutputFuzzySetMessage=warning
  Mux : Mux  Inputs=2
  Product : Product  OutDataTypeStr=int16
  Saturation : Saturate  UpperLimit=100  LowerLimit=0  OutDataTypeStr=int16
  Saturation1 : Saturate  UpperLimit=300  LowerLimit=-300  OutDataTypeStr=int16
  Saturation2 : Saturate  UpperLimit=100  LowerLimit=0  OutDataTypeStr=int16
  Subtract1 : Sum  Inputs=+-  OutDataTypeStr=int16
  Variable Integer Delay : Delay  DelayLengthSource=Input port
      settings: InputPortMap=u0,p1
  Inten : Outport  VectorParamsAs1DForOutWhenUnconnected=off
  wires:
  Subtract1/1 -> Product/1
  Constant2/1 -> Divide/2
  Constant1/1 -> Divide/1, Divide1/2
  Divide1/1 -> Product/2
  Divide/1 -> Variable Integer Delay/2
  Variable Integer Delay/1 -> Subtract1/2
  Saturation/1 -> Mux/1
  Fuzzy Logic Controller/1 -> Saturation2/1
  Constant3/1 -> Divide1/1
  Mux/1 -> Fuzzy Logic Controller/1
  Saturation1/1 -> Mux/2
  AccPeld/1 -> Subtract1/1, Variable Integer Delay/1, Saturation/1
  Product/1 -> Saturation1/1
  Saturation2/1 -> Inten/1

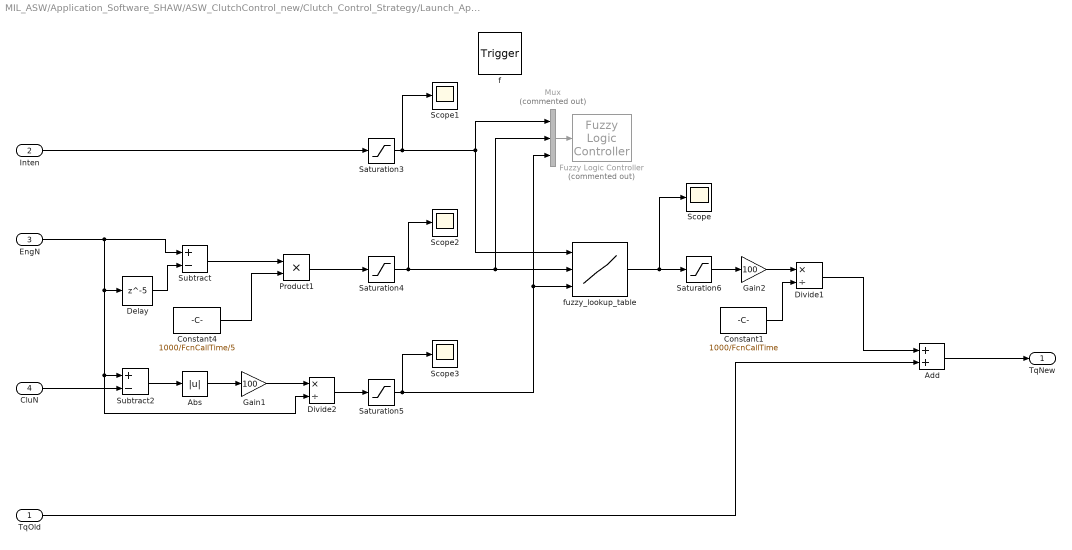
== system MIL_ASW/Application_Software_SHAW/ASW_ClutchControl_new/Clutch_Control_Strategy/Launch_Applied_Fuzzy ==
  TqOld : Inport  OutDataTypeStr=uint16  PortDimensions=1
  Inten : Inport  Port=2  OutDataTypeStr=int16  PortDimensions=1
  EngN : Inport  Port=3  OutDataTypeStr=int16  PortDimensions=1
  CluN : Inport  Port=4  OutDataTypeStr=int16  PortDimensions=1
  f : TriggerPort  TriggerType=function-call  VariantControl=(inherit)
      settings: CopyFcn=Stateflow.SLINSF.SimulinkMan.removeBlockPreDeleteFcn  PreDeleteFcn=Stateflow.SLINSF.SimulinkMan.unsafePredeleteFcn
  Abs : Abs
  Add : Sum  OutDataTypeStr=uint16
  Constant1 : Constant  Value=1000/FcnCallTime  OutDataTypeStr=uint16
  Constant4 : Constant  Value=1000/FcnCallTime/5  OutDataTypeStr=int16
  Delay : Delay  DelayLength=5
  Divide1 : Product  Inputs=*/  OutDataTypeStr=uint16
  Divide2 : Product  Inputs=*/  OutDataTypeStr=int16
  Fuzzy Logic Controller : fuzblock/Fuzzy Logic  Controller  Commented=on  FIS='Launch_Engage_Fuzzy.fis'  OutputSampleNumber=101  DataType=single  FuzzifiedInputs=off  RuleFiringStrengths=off  RuleOutputs=off  AggregatedOutputs=off  SimulateUsing=Interpreted execution  OutOfRangeInputValueMessage=warning  NoRuleFiredMessage=warning  EmptyOutputFuzzySetMessage=warning
  Gain1 : Gain  Gain=100
  Gain2 : Gain  Gain=100
  Mux : Mux  Commented=on  Inputs=3
  Product1 : Product  OutDataTypeStr=int16
  Saturation3 : Saturate  UpperLimit=100  LowerLimit=0  OutDataTypeStr=int16
  Saturation4 : Saturate  UpperLimit=1000  LowerLimit=-1000  OutDataTypeStr=int16
  Saturation5 : Saturate  UpperLimit=100  LowerLimit=0  OutDataTypeStr=int16
  Saturation6 : Saturate  UpperLimit=350  LowerLimit=0  OutDataTypeStr=uint16
  Scope{,1..3} (4 alike) : Scope
  Subtract : Sum  Inputs=+-  OutDataTypeStr=int16
  Subtract2 : Sum  Inputs=+-  OutDataTypeStr=int16
  fuzzy_lookup_table : Lookup_n-D  NumberOfTableDimensions=3  DataSpecification=Lookup table object  LookupTableObject=LnchEngmtFzzy  BreakpointsForDimension1=in1  BreakpointsForDimension2=in1  BreakpointsForDimension1DataTypeStr=int16  BreakpointsForDimension2DataTypeStr=int16  Table=out1  TableDataTypeStr=int16  ExtrapMethod=Clip  UseLastTableValue=on  InternalRulePriority=Speed  OutDataTypeStr=Inherit: Inherit from 'Table data'  RndMeth=Simplest  InputSameDT=on
  TqNew : Outport  OutDataTypeStr=uint16  VectorParamsAs1DForOutWhenUnconnected=off
  wires:
  Delay/1 -> Subtract/2
  CluN/1 -> Subtract2/2
  Saturation3/1 -> Scope1/1, Mux/1, fuzzy_lookup_table/1
  Abs/1 -> Gain1/1
  Gain1/1 -> Divide2/1
  Subtract2/1 -> Abs/1
  Subtract/1 -> Product1/1
  Constant4/1 -> Product1/2
  Saturation5/1 -> Scope3/1, Mux/3, fuzzy_lookup_table/3
  EngN/1 -> Delay/1, Subtract2/1, Divide2/2, Subtract/1
  Saturation4/1 -> Scope2/1, Mux/2, fuzzy_lookup_table/2
  Divide2/1 -> Saturation5/1
  Inten/1 -> Saturation3/1
  fuzzy_lookup_table/1 -> Scope/1, Saturation6/1
  Saturation6/1 -> Gain2/1
  TqOld/1 -> Add/2
  Add/1 -> TqNew/1
  Gain2/1 -> Divide1/1
  Constant1/1 -> Divide1/2
  Divide1/1 -> Add/1
  Mux/1 -> Fuzzy Logic Controller/1
  Product1/1 -> Saturation4/1
